simulink subsystem "decision_making"  (R2022b)
settings: Solver=VariableStepAuto  StartTime=0.0  StopTime=10.0  RelTol=1e-3
libraries: simulink x7, dspstat3 x4, slpidlib x1
settings Model: Creator=micha  LastModifiedBy=adter
settings ModelReferenceCC: EnableRefExpFcnMdlSchedulingChecks=on

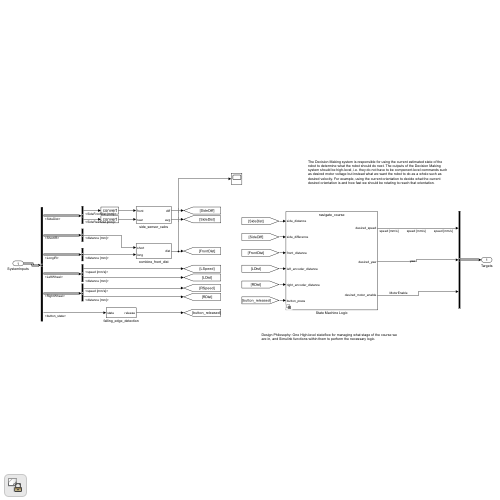
[thumbnail: Simulink's stored preview of the top-level diagram]
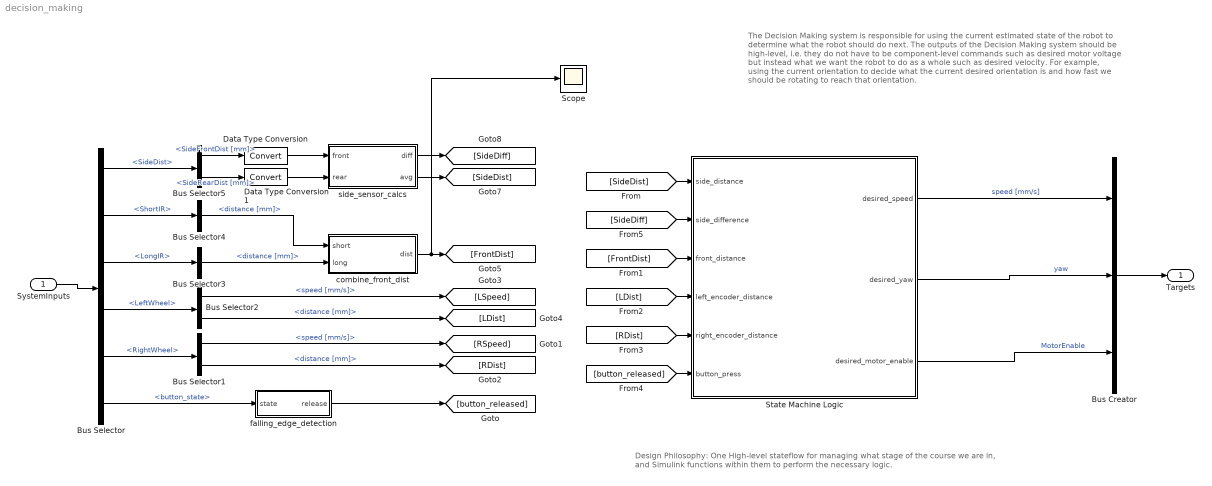
== system decision_making ==
  note: Design Philosophy: One High-level stateflow for managing what stage of the course we are in, and Simulink functions within them to perform the necessary logic.
  note: The Decision Making system is responsible for using the current estimated state of the robot to determine what the robot should do next. The outputs of the Decision Making system should be high-level, i.e. they do not have to be component-level commands such as desired motor voltage but instead what we want the robot to do as a whole such as desired velocity. For example, using the current orientation to decide what the current desired orientation is and how fast we should be rotating to reach that orientation.
  SystemInputs : Inport
  Bus Creator : BusCreator  Inputs=3
  Bus Selector : BusSelector  OutputSignals=SideDist,ShortIR,LongIR,LeftWheel,RightWheel,button.button_state
  Bus Selector1 : BusSelector  OutputSignals=speed [mm/s],distance [mm]
  Bus Selector2 : BusSelector  OutputSignals=speed [mm/s],distance [mm]
  Bus Selector3 : BusSelector  OutputSignals=distance [mm]
  Bus Selector4 : BusSelector  OutputSignals=distance [mm]
  Bus Selector5 : BusSelector  OutputSignals=SideFrontDist [mm],SideRearDist [mm]
  Data Type Conversion : DataTypeConversion  SaturateOnIntegerOverflow=off  RndMeth=Floor
  Data Type Conversion1 : DataTypeConversion  SaturateOnIntegerOverflow=off  RndMeth=Floor
  Scope : Scope
  State Machine Logic : Subsystem  Variant=on  VariantControlMode=label  LabelModeActiveChoice=true
  combine_front_dist : Subsystem
  falling_edge_detection : Subsystem
  side_sensor_calcs : Subsystem
  Targets : Outport
  wires:
  SystemInputs/1 -> Bus Selector/1
  State Machine Logic/2(desired_yaw) -> Bus Creator/2  "yaw"
  Bus Creator/1 -> Targets/1
  State Machine Logic/3(desired_motor_enable) -> Bus Creator/3  "MotorEnable"
  Bus Selector/6 -> falling_edge_detection/1(state)  "<button_state>"
  falling_edge_detection/1(release) -> [button_released]
  Bus Selector/5 -> Bus Selector1/1  "<RightWheel>"
  Bus Selector1/1 -> [RSpeed]  "<speed [mm/s]>"
  Bus Selector1/2 -> [RDist]  "<distance [mm]>"
  Bus Selector2/2 -> [LDist]  "<distance [mm]>"
  Bus Selector2/1 -> [LSpeed]  "<speed [mm/s]>"
  Bus Selector/4 -> Bus Selector2/1  "<LeftWheel>"
  Bus Selector/2 -> Bus Selector4/1  "<ShortIR>"
  Bus Selector/3 -> Bus Selector3/1  "<LongIR>"
  Bus Selector3/1 -> combine_front_dist/2(long)  "<distance [mm]>"
  Bus Selector4/1 -> combine_front_dist/1(short)  "<distance [mm]>"
  combine_front_dist/1(dist) -> [FrontDist], Scope/1
  [SideDist] -> State Machine Logic/1(side_distance)
  [FrontDist] -> State Machine Logic/3(front_distance)
  [LDist] -> State Machine Logic/4(left_encoder_distance)
  [RDist] -> State Machine Logic/5(right_encoder_distance)
  [button_released] -> State Machine Logic/6(button_press)
  State Machine Logic/1(desired_speed) -> Bus Creator/1  "speed [mm/s]"
  Bus Selector/1 -> Bus Selector5/1  "<SideDist>"
  Bus Selector5/2 -> Data Type Conversion1/1  "<SideRearDist [mm]>"
  Bus Selector5/1 -> Data Type Conversion/1  "<SideFrontDist [mm]>"
  side_sensor_calcs/2(avg) -> [SideDist]
  side_sensor_calcs/1(diff) -> [SideDiff]
  [SideDiff] -> State Machine Logic/2(side_difference)
  Data Type Conversion/1 -> side_sensor_calcs/1(front)
  Data Type Conversion1/1 -> side_sensor_calcs/2(rear)

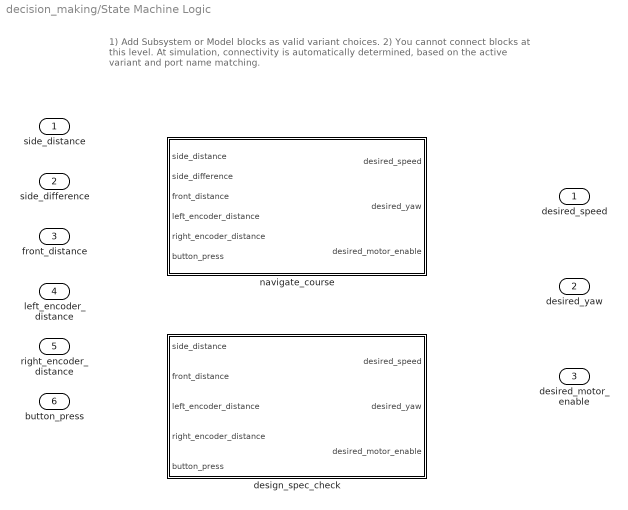
== system decision_making/State Machine Logic ==
  note: 1) Add Subsystem or Model blocks as valid variant choices.
      | 2) You cannot connect blocks at this level. At simulation, connectivity is automatically
      | determined, based on the active variant and port name matching.
  side_distance : Inport
  side_difference : Inport  Port=2
  front_distance : Inport  Port=3
  left_encoder_distance : Inport  Port=4
  right_encoder_distance : Inport  Port=5
  button_press : Inport  Port=6
  design_spec_check : Subsystem  VariantControl=false
  navigate_course : Subsystem  VariantControl=true
  desired_speed : Outport
  desired_yaw : Outport  Port=2
  desired_motor_enable : Outport  Port=3

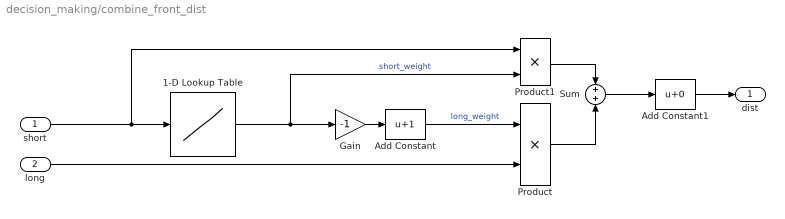
== system decision_making/combine_front_dist ==
  short : Inport
  long : Inport  Port=2
  1-D Lookup Table : Lookup_n-D  NumberOfTableDimensions=1  BreakpointsForDimension1=[0, 150, 300, 1000]  Table=[1, 1, 0, 0]  InternalRulePriority=Speed  RndMeth=Simplest
  Add Constant : Bias  Bias=1  SaturateOnIntegerOverflow=off
  Add Constant1 : Bias  SaturateOnIntegerOverflow=off
  Gain : Gain  Gain=-1
  Product : Product
  Product1 : Product
  Sum : Sum
  dist : Outport
  wires:
  Add Constant1/1 -> dist/1
  Sum/1 -> Add Constant1/1
  Product1/1 -> Sum/1
  Product/1 -> Sum/2
  long/1 -> Product/2
  Add Constant/1 -> Product/1  "long_weight"
  Gain/1 -> Add Constant/1
  1-D Lookup Table/1 -> Gain/1, Product1/2  "short_weight"
  short/1 -> 1-D Lookup Table/1, Product1/1

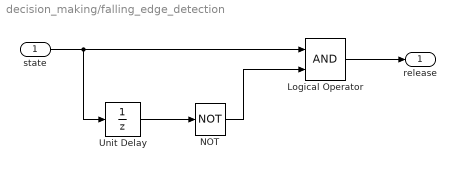
== system decision_making/falling_edge_detection ==
  state : Inport
  Logical Operator : Logic  IconShape=distinctive  AllPortsSameDT=off  OutDataTypeStr=boolean
  NOT : Logic  Operator=NOT  IconShape=distinctive  AllPortsSameDT=off  OutDataTypeStr=boolean
  Unit Delay : UnitDelay  SampleTime=-1  HasFrameUpgradeWarning=on
  release : Outport
  wires:
  NOT/1 -> Logical Operator/2
  state/1 -> Unit Delay/1, Logical Operator/1
  Logical Operator/1 -> release/1
  Unit Delay/1 -> NOT/1

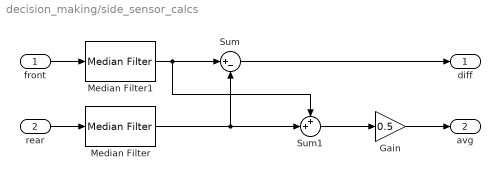
== system decision_making/side_sensor_calcs ==
  front : Inport
  rear : Inport  Port=2
  Gain : Gain  Gain=0.5
  Median Filter : dspstat3/Median Filter  WindowLength=5  SimulateUsing=Code generation
      settings: LibrarySourceBlock=|
      | dspfdesign/Median
      | Filter
  Median Filter1 : dspstat3/Median Filter  WindowLength=5  SimulateUsing=Code generation
      settings: LibrarySourceBlock=|
      | dspfdesign/Median
      | Filter
  Sum : Sum  Inputs=|+-
  Sum1 : Sum  Inputs=++|
  diff : Outport
  avg : Outport  Port=2
  wires:
  Median Filter1/1 -> Sum/1, Sum1/1
  Median Filter/1 -> Sum/2, Sum1/2
  Gain/1 -> avg/1
  Sum1/1 -> Gain/1
  Sum/1 -> diff/1
  rear/1 -> Median Filter/1
  front/1 -> Median Filter1/1

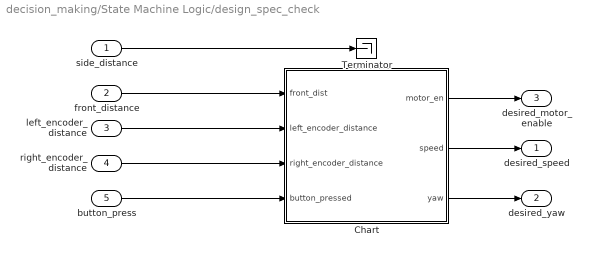
== system decision_making/State Machine Logic/design_spec_check ==
  side_distance : Inport
  front_distance : Inport  Port=2
  left_encoder_distance : Inport  Port=3
  right_encoder_distance : Inport  Port=4
  button_press : Inport  Port=5
  Chart : Stateflow chart  TreatAsAtomicUnit=on
  Terminator : Terminator
  desired_speed : Outport
  desired_yaw : Outport  Port=2
  desired_motor_enable : Outport  Port=3
  wires:
  button_press/1 -> Chart/4(button_pressed)
  front_distance/1 -> Chart/1(front_dist)
  right_encoder_distance/1 -> Chart/3(right_encoder_distance)
  left_encoder_distance/1 -> Chart/2(left_encoder_distance)
  side_distance/1 -> Terminator/1
  Chart/2(speed) -> desired_speed/1
  Chart/3(yaw) -> desired_yaw/1
  Chart/1(motor_en) -> desired_motor_enable/1

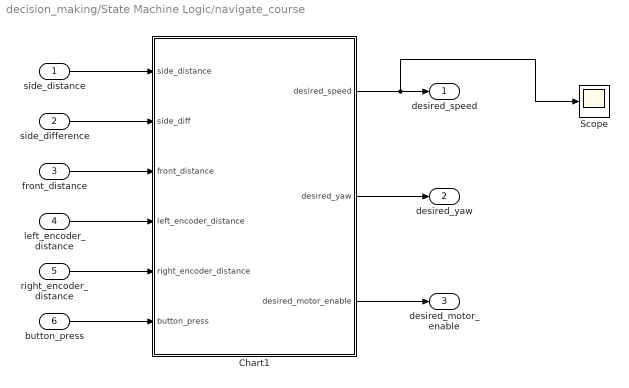
== system decision_making/State Machine Logic/navigate_course ==
  side_distance : Inport
  side_difference : Inport  Port=2
  front_distance : Inport  Port=3
  left_encoder_distance : Inport  Port=4
  right_encoder_distance : Inport  Port=5
  button_press : Inport  Port=6
  Chart1 : Stateflow chart  TreatAsAtomicUnit=on
  Scope : Scope
  desired_speed : Outport
  desired_yaw : Outport  Port=2
  desired_motor_enable : Outport  Port=3
  wires:
  side_difference/1 -> Chart1/2(side_diff)
  Chart1/3(desired_motor_enable) -> desired_motor_enable/1
  Chart1/2(desired_yaw) -> desired_yaw/1
  Chart1/1(desired_speed) -> desired_speed/1, Scope/1
  button_press/1 -> Chart1/6(button_press)
  right_encoder_distance/1 -> Chart1/5(right_encoder_distance)
  left_encoder_distance/1 -> Chart1/4(left_encoder_distance)
  front_distance/1 -> Chart1/3(front_distance)
  side_distance/1 -> Chart1/1(side_distance)

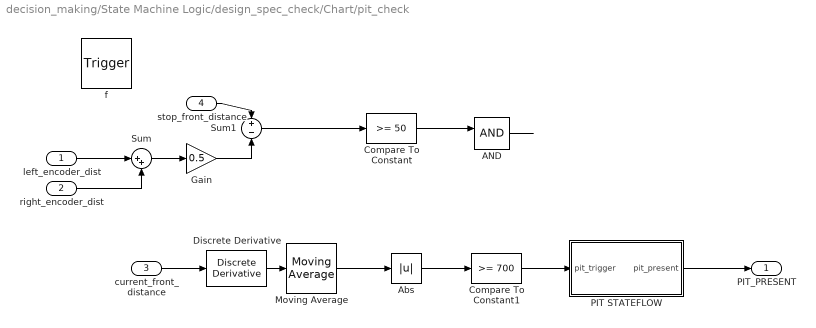
== system decision_making/State Machine Logic/design_spec_check/Chart/pit_check ==
  left_encoder_dist : Inport  OutDataTypeStr=int64  PortDimensions=1
  right_encoder_dist : Inport  Port=2  OutDataTypeStr=int64  PortDimensions=1
  current_front_distance : Inport  Port=3  OutDataTypeStr=double  PortDimensions=1
  stop_front_distance : Inport  Port=4  OutDataTypeStr=double  PortDimensions=1
  f : TriggerPort  TriggerType=function-call  VariantControl=(inherit)
      settings: CopyFcn=Stateflow.SLINSF.SimulinkMan.removeBlockPreDeleteFcn  PreDeleteFcn=Stateflow.SLINSF.SimulinkMan.unsafePredeleteFcn
  AND : Logic  IconShape=distinctive  AllPortsSameDT=off  OutDataTypeStr=boolean
  Abs : Abs  SaturateOnIntegerOverflow=off
  Compare To Constant : simulink/Logic and Bit Operations/Compare To Constant  relop=>=  const=50  OutDataTypeStr=boolean
  Compare To Constant1 : simulink/Logic and Bit Operations/Compare To Constant  relop=>=  const=700  OutDataTypeStr=boolean
  Discrete Derivative : simulink/Discrete/Discrete Derivative  gainval=1.0  ICPrevScaledInput=0.0  OutMin=[]  OutMax=[]  OutDataType=fixdt(1, 16)  OutScaling=2^-10  DoSatur=off
  Gain : Gain  Gain=0.5
  Moving Average : dspstat3/Moving Average  Method=Sliding window  ForgettingFactorPort=off  SpecifyWindowLength=on  WindowLength=50  OverlapLength=49  AllowArbitraryInputLength=off  ForgettingFactor=0.9  SimulateUsing=Code generation
  PIT STATEFLOW : Stateflow chart  TreatAsAtomicUnit=on
  Sum : Sum  Inputs=|++
  Sum1 : Sum  Inputs=+|-
  PIT_PRESENT : Outport  OutDataTypeStr=boolean
  wires:
  Abs/1 -> Compare To Constant1/1
  AND/1 -> ?
  PIT STATEFLOW/1(pit_present) -> PIT_PRESENT/1
  Compare To Constant/1 -> AND/1
  Moving Average/1 -> Abs/1
  Discrete Derivative/1 -> Moving Average/1
  Compare To Constant1/1 -> PIT STATEFLOW/1(pit_trigger)
  current_front_distance/1 -> Discrete Derivative/1
  Sum1/1 -> Compare To Constant/1
  Gain/1 -> Sum1/2
  stop_front_distance/1 -> Sum1/1
  Sum/1 -> Gain/1
  left_encoder_dist/1 -> Sum/1
  right_encoder_dist/1 -> Sum/2

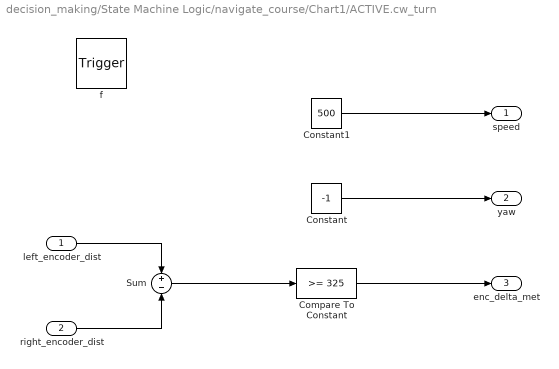
== system decision_making/State Machine Logic/navigate_course/Chart1/ACTIVE.cw_turn ==
  left_encoder_dist : Inport  OutDataTypeStr=int64  PortDimensions=1
  right_encoder_dist : Inport  Port=2  OutDataTypeStr=int64  PortDimensions=1
  f : TriggerPort  TriggerType=function-call  VariantControl=(inherit)
      settings: CopyFcn=Stateflow.SLINSF.SimulinkMan.removeBlockPreDeleteFcn  PreDeleteFcn=Stateflow.SLINSF.SimulinkMan.unsafePredeleteFcn
  Compare To Constant : simulink/Logic and Bit Operations/Compare To Constant  relop=>=  const=325  OutDataTypeStr=boolean
  Constant : Constant  Value=-1
  Constant1 : Constant  Value=500
  Sum : Sum  Inputs=+|-
  speed : Outport  OutDataTypeStr=double
  yaw : Outport  Port=2  OutDataTypeStr=double
  enc_delta_met : Outport  Port=3
  wires:
  Sum/1 -> Compare To Constant/1
  Compare To Constant/1 -> enc_delta_met/1
  right_encoder_dist/1 -> Sum/2
  left_encoder_dist/1 -> Sum/1
  Constant1/1 -> speed/1
  Constant/1 -> yaw/1

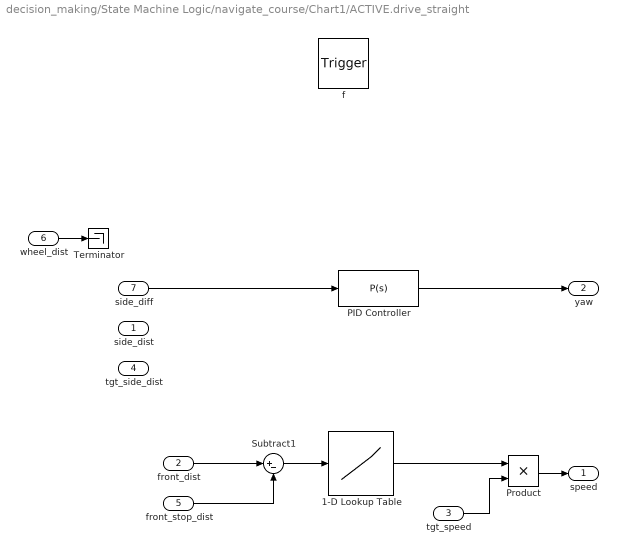
== system decision_making/State Machine Logic/navigate_course/Chart1/ACTIVE.drive_straight ==
  side_dist : Inport  OutDataTypeStr=double  PortDimensions=1
  front_dist : Inport  Port=2  OutDataTypeStr=double  PortDimensions=1
  tgt_speed : Inport  Port=3  OutDataTypeStr=double  PortDimensions=1
  tgt_side_dist : Inport  Port=4  OutDataTypeStr=double  PortDimensions=1
  front_stop_dist : Inport  Port=5  OutDataTypeStr=double  PortDimensions=1
  wheel_dist : Inport  Port=6  OutDataTypeStr=int64  PortDimensions=1
  side_diff : Inport  Port=7  OutDataTypeStr=double  PortDimensions=1
  f : TriggerPort  TriggerType=function-call  VariantControl=(inherit)  SampleTimeType=periodic  SampleTime=(-1)
      settings: CopyFcn=Stateflow.SLINSF.SimulinkMan.removeBlockPreDeleteFcn  PreDeleteFcn=Stateflow.SLINSF.SimulinkMan.unsafePredeleteFcn
  1-D Lookup Table : Lookup_n-D  NumberOfTableDimensions=1  BreakpointsForDimension1=[0,150,2000]  Table=[0.1,1,1]  ExtrapMethod=Clip  UseLastTableValue=on  InternalRulePriority=Speed  RndMeth=Simplest
  PID Controller : slpidlib/PID Controller  Controller=P  Form=Parallel  TimeDomain=Continuous-time  UseExternalTs=off  SampleTime=-1  IntegratorMethod=Forward Euler  FilterMethod=Forward Euler  ControllerParametersSource=internal  P=0.25/20  I=1  UseKiTs=off  D=0  N=100  UseFilter=on  TunerSelectOption=Transfer Function Based (PID Tuner App)  InitialConditionSource=internal  InitialConditionForIntegrator=0  InitialConditionForFilter=0  DifferentiatorICPrevScaledInput=0  ExternalReset=none  TrackingMode=off  Kt=1  LimitOutput=on  SatLimitsSource=internal  UpperSaturationLimit=0.25  LowerSaturationLimit=-0.25  LinearizeAsGain=on  AntiWindupMode=none  Kb=1  LimitIntegrator=off  UpperIntegratorSaturationLimit=inf  LowerIntegratorSaturationLimit=-inf  POutMin=[]  POutMax=[]  IOutMin=[]  IOutMax=[]  DOutMin=[]  DOutMax=[]  NOutMin=[]  NOutMax=[]  SumOutMin=[]  SumOutMax=[]  SaturationOutMin=[]  SaturationOutMax=[]  PParamMin=[]  PParamMax=[]  IParamMin=[]  IParamMax=[]  DParamMin=[]  DParamMax=[]  NParamMin=[]  NParamMax=[]  KbParamMin=[]  KbParamMax=[]  KtParamMin=[]  KtParamMax=[]  KbOutMin=[]  KbOutMax=[]  KtOutMin=[]  KtOutMax=[]  IntegratorOutMin=[]  IntegratorOutMax=[]  FilterOutMin=[]  FilterOutMax=[]  SumI1OutMin=[]  SumI1OutMax=[]  SumI2OutMin=[]  SumI2OutMax=[]  SumI3OutMin=[]  SumI3OutMax=[]  SumI4OutMin=[]  SumI4OutMax=[]  SumDOutMin=[]  SumDOutMax=[]  DifferentiatorOutMin=[]  DifferentiatorOutMax=[]  FilterDiffOutCoefMin=[]  FilterDiffOutCoefMax=[]  ReciprocalOutMin=[]  ReciprocalOutMax=[]  SumDenOutMin=[]  SumDenOutMax=[]  SumNumOutMin=[]  SumNumOutMax=[]  DivideOutMin=[]  DivideOutMax=[]  UdiffTsProdOutMin=[]  UdiffTsProdOutMax=[]  NTsProdOutMin=[]  NTsProdOutMax=[]  UintegralTsProdOutMin=[]  UintegralTsProdOutMax=[]  UngainTsProdOutMin=[]  UngainTsProdOutMax=[]  ClampingZeroOutDataTypeStr=Inherit: Inherit via back propagation  ClampingZeroOutMin=[]  ClampingZeroOutMax=[]  FilterDenConstantOutDataTypeStr=Inherit: Inherit via back propagation  FilterDenConstantOutMin=[]  FilterDenConstantOutMax=[]  PCopyOutDataTypeStr=Inherit: Inherit via back propagation  PCopyOutMin=[]  PCopyOutMax=[]  NCopyOutDataTypeStr=Inherit: Inherit via back propagation  NCopyOutMin=[]  NCopyOutMax=[]  IntegratorContinuousStateAttributes=''  IntegratorStateMustResolveToSignalObject=off  IntegratorRTWStateStorageClass=Auto  FilterContinuousStateAttributes=''  FilterStateMustResolveToSignalObject=off  FilterRTWStateStorageClass=Auto  ParallelPVariant=InternalParameters  IdealPVariant=Disabled  IVariant=Disabled  DVariant=Disabled  IntegratorVariant=Disabled  SatVariant=Enabled  AWVariant=Disabled  PCopyVariant=Disabled  TRVariant=Disabled  FdbkBlocksVariant=Forward  IdealPFdbkVariant=Disabled  SatFdbkVariant=Disabled  DerivativeFilterVariant=Disabled  NVariant=Disabled  NCopyVariant=Disabled_SignalSpec  FilterICVariant=Disabled  IntegratorICVariant=Disabled  ExternalResetVariant=Disabled  TRSumVariant=Passthrough  SumFdbkVariant=Disabled  SumVariant=Passthrough_P  TsampFilterVariant=InternalTs  TsampNgainVariant=Passthrough  TsampIntegralVariant=Disabled_SignalSpec  ExternalSaturationOutDataTypeStr=Inherit: Same as second input
  Product : Product
  Subtract1 : Sum  Inputs=|+-
  Terminator : Terminator
  speed : Outport
  yaw : Outport  Port=2
  wires:
  PID Controller/1 -> yaw/1
  side_diff/1 -> PID Controller/1
  Product/1 -> speed/1
  wheel_dist/1 -> Terminator/1
  tgt_speed/1 -> Product/2
  1-D Lookup Table/1 -> Product/1
  front_stop_dist/1 -> Subtract1/2
  front_dist/1 -> Subtract1/1
  Subtract1/1 -> 1-D Lookup Table/1

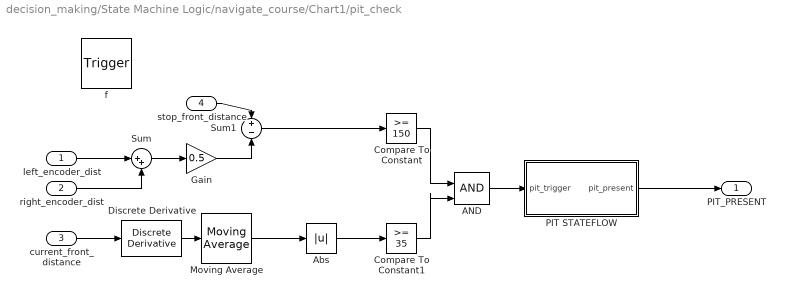
== system decision_making/State Machine Logic/navigate_course/Chart1/pit_check ==
  left_encoder_dist : Inport  OutDataTypeStr=int64  PortDimensions=1
  right_encoder_dist : Inport  Port=2  OutDataTypeStr=int64  PortDimensions=1
  current_front_distance : Inport  Port=3  OutDataTypeStr=double  PortDimensions=1
  stop_front_distance : Inport  Port=4  OutDataTypeStr=double  PortDimensions=1
  f : TriggerPort  TriggerType=function-call  VariantControl=(inherit)
      settings: CopyFcn=Stateflow.SLINSF.SimulinkMan.removeBlockPreDeleteFcn  PreDeleteFcn=Stateflow.SLINSF.SimulinkMan.unsafePredeleteFcn
  AND : Logic  IconShape=distinctive  AllPortsSameDT=off  OutDataTypeStr=boolean
  Abs : Abs  SaturateOnIntegerOverflow=off
  Compare To Constant : simulink/Logic and Bit Operations/Compare To Constant  relop=>=  const=150  OutDataTypeStr=boolean
  Compare To Constant1 : simulink/Logic and Bit Operations/Compare To Constant  relop=>=  const=35  OutDataTypeStr=boolean
  Discrete Derivative : simulink/Discrete/Discrete Derivative  gainval=1.0  ICPrevScaledInput=0.0  OutMin=[]  OutMax=[]  OutDataType=fixdt(1, 16)  OutScaling=2^-10  DoSatur=off
  Gain : Gain  Gain=0.5
  Moving Average : dspstat3/Moving Average  Method=Sliding window  ForgettingFactorPort=off  SpecifyWindowLength=on  WindowLength=50  OverlapLength=49  AllowArbitraryInputLength=off  ForgettingFactor=0.9  SimulateUsing=Code generation
  PIT STATEFLOW : Stateflow chart  TreatAsAtomicUnit=on
  Sum : Sum  Inputs=|++
  Sum1 : Sum  Inputs=+|-
  PIT_PRESENT : Outport  OutDataTypeStr=boolean
  wires:
  Abs/1 -> Compare To Constant1/1
  AND/1 -> PIT STATEFLOW/1(pit_trigger)
  PIT STATEFLOW/1(pit_present) -> PIT_PRESENT/1
  Compare To Constant/1 -> AND/1
  Moving Average/1 -> Abs/1
  Discrete Derivative/1 -> Moving Average/1
  Compare To Constant1/1 -> AND/2
  current_front_distance/1 -> Discrete Derivative/1
  Sum1/1 -> Compare To Constant/1
  Gain/1 -> Sum1/2
  stop_front_distance/1 -> Sum1/1
  Sum/1 -> Gain/1
  left_encoder_dist/1 -> Sum/1
  right_encoder_dist/1 -> Sum/2

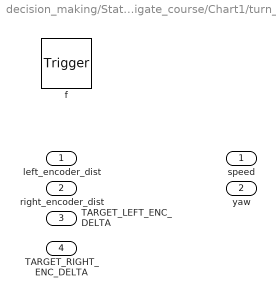
== system decision_making/State Machine Logic/navigate_course/Chart1/turn_zero ==
  left_encoder_dist : Inport  OutDataTypeStr=double  PortDimensions=1
  right_encoder_dist : Inport  Port=2  OutDataTypeStr=double  PortDimensions=1
  TARGET_LEFT_ENC_DELTA : Inport  Port=3  OutDataTypeStr=double  PortDimensions=1
  TARGET_RIGHT_ENC_DELTA : Inport  Port=4  OutDataTypeStr=double  PortDimensions=1
  f : TriggerPort  TriggerType=function-call  VariantControl=(inherit)
      settings: CopyFcn=Stateflow.SLINSF.SimulinkMan.removeBlockPreDeleteFcn  PreDeleteFcn=Stateflow.SLINSF.SimulinkMan.unsafePredeleteFcn
  speed : Outport
  yaw : Outport  Port=2

== stateflow chart decision_making/State Machine Logic/navigate_course/Chart1/pit_check/PIT STATEFLOW ==
  state OUT_OF_PIT
    en: pit_present = false;
  state IN_PIT
    en: pit_present = true;
    en: pit_time = et;
  (default) -> OUT_OF_PIT
  IN_PIT -> OUT_OF_PIT : [pit_trigger == true && (pit_time - et) > 0.5]
  OUT_OF_PIT -> IN_PIT : [pit_trigger == true]
  data: pit_trigger input boolean; pit_present output boolean =false; pit_time local =0

== stateflow chart decision_making/State Machine Logic/design_spec_check/Chart ==
  state IDLE
    en, du: motor_en = false;
    en, du: speed = 0;
    en, du: yaw = 0;
    du: [pit_detected] = pit_check(left_encoder_distance, right_encoder_distance, front_dist, STOP_DIST);
  state PIT_PRESENT  = pit_check(left_encoder_dist,right_encoder_dist, current_front_distance, stop_front_distance) [function]
  state TEST1
    en, du: motor_en = true;
    en, du: yaw = 0;
    en, du: speed = 600;
    du: [pit_detected] = pit_check(left_encoder_distance, right_encoder_distance, front_dist, STOP_DIST);
  state TEST3
    en, du: motor_en = true;
    en, du: yaw = 0;
    en, du: speed = 200;
    du: [pit_detected] = pit_check(left_encoder_distance, right_encoder_distance, front_dist, STOP_DIST);
  (default) -> IDLE
  TEST3 -> IDLE : [button_pressed || front_dist <= STOP_DIST]
  TEST1 -> IDLE [order 1] : [button_pressed || front_dist <= STOP_DIST]
  IDLE -> TEST1 : [button_pressed]
  TEST1 -> TEST3 [order 2] : [pit_detected]
  data: left_encoder_dist function_input int64 size=1; right_encoder_dist function_input int64 size=1; PIT_PRESENT function_output boolean; current_front_distance function_input double size=1; stop_front_distance function_input double size=1; motor_en output boolean; speed output; yaw output; STOP_DIST constant double =100; front_dist input; left_encoder_distance input; right_encoder_distance input; button_pressed input boolean; pit_detected local

== stateflow chart decision_making/State Machine Logic/navigate_course/Chart1 ==
  state PIT_PRESENT  = pit_check(left_encoder_dist,right_encoder_dist, current_front_distance, stop_front_distance) [function] [commented out]
  state IDLE
    en: desired_speed = 0;
    en: desired_yaw = 0;
    en: desired_motor_enable = false;
  state [speed, yaw] =   turn_zero(left_encoder_dist, right_encoder_dist, TARGET_LEFT_ENC_DELTA, TARGET_RIGHT_ENC_DELTA) [function] [commented out]
  state ACTIVE
    en: desired_motor_enable = true;
    state [speed,yaw] = drive_straight(side_dist,front_dist,tgt_speed,tgt_side_dist,front_stop_dist,wheel_dist,side_diff) [function]
    state [speed,yaw,enc_delta_met] = cw_turn(left_encoder_dist,right_encoder_dist) [function]
    state STAGE_0_DRIVE
      en: left_eref = left_encoder_distance;
      en: right_eref = right_encoder_distance;
      en,during: [desired_speed, desired_yaw] = drive_straight(side_distance, front_distance, TARGET_SPEED, OUTER_LOOP_SIDE_DIST,...
      OUTER_LOOP_FRONT_STOP_DIST, ((left_encoder_distance - left_eref) + (right_encoder_distance - right_eref))/2, side_diff);
    state STAGE_0_TURN
      en: ENC_DELTAS_MET = false;
      en: left_eref = left_encoder_distance;
      en: right_eref = right_encoder_distance;
      en: in_pit = false;
      du: [desired_speed, desired_yaw, ENC_DELTAS_MET] = cw_turn((left_encoder_distance - left_eref), (right_encoder_distance - right_eref));
    state STAGE_1_DRIVE
      en: left_eref = left_encoder_distance;
      en: right_eref = right_encoder_distance;
      en,during: [desired_speed, desired_yaw] = drive_straight(side_distance, front_distance, TARGET_SPEED, OUTER_LOOP_SIDE_DIST,...
      OUTER_LOOP_FRONT_STOP_DIST, ((left_encoder_distance - left_eref) + (right_encoder_distance - right_eref))/2, side_diff);
    state STAGE_1_TURN
      en: ENC_DELTAS_MET = false;
      en: left_eref = left_encoder_distance;
      en: right_eref = right_encoder_distance;
      en: in_pit = false;
      du: [desired_speed, desired_yaw, ENC_DELTAS_MET] = cw_turn((left_encoder_distance - left_eref), (right_encoder_distance - right_eref));
    state STAGE_2_DRIVE
      en: left_eref = left_encoder_distance;
      en: right_eref = right_encoder_distance;
      en,during: [desired_speed, desired_yaw] = drive_straight(side_distance, front_distance, TARGET_SPEED, OUTER_LOOP_SIDE_DIST,...
      OUTER_LOOP_FRONT_STOP_DIST, ((left_encoder_distance - left_eref) + (right_encoder_distance - right_eref))/2, side_diff);
    state STAGE_2_TURN
      en: ENC_DELTAS_MET = false;
      en: left_eref = left_encoder_distance;
      en: right_eref = right_encoder_distance;
      en: in_pit = false;
      du: [desired_speed, desired_yaw, ENC_DELTAS_MET] = cw_turn((left_encoder_distance - left_eref), (right_encoder_distance - right_eref));
    state STAGE_3_DRIVE
      en: left_eref = left_encoder_distance;
      en: right_eref = right_encoder_distance;
      en,during: [desired_speed, desired_yaw] = drive_straight(side_distance, front_distance, TARGET_SPEED, MIDDLE_LOOP_SIDE_DIST,...
      MIDDLE_LOOP_FRONT_STOP_DIST, ((left_encoder_distance - left_eref) + (right_encoder_distance - right_eref))/2, side_diff);
    state STAGE_3_TURN
      en: ENC_DELTAS_MET = false;
      en: left_eref = left_encoder_distance;
      en: right_eref = right_encoder_distance;
      en: in_pit = false;
      du: [desired_speed, desired_yaw, ENC_DELTAS_MET] = cw_turn((left_encoder_distance - left_eref), (right_encoder_distance - right_eref));
    (default) -> STAGE_0_DRIVE
    STAGE_0_DRIVE -> STAGE_0_TURN [order 1] : [front_distance <= OUTER_LOOP_FRONT_STOP_DIST &&...
        | ((left_encoder_distance - left_eref) + (right_encoder_distance - right_eref))/2 > 500]
    STAGE_0_TURN -> STAGE_1_DRIVE : [ENC_DELTAS_MET]
    STAGE_1_DRIVE -> STAGE_1_TURN : [front_distance <= OUTER_LOOP_FRONT_STOP_DIST &&...
        | ((left_encoder_distance - left_eref) + (right_encoder_distance - right_eref))/2 > 500]
    STAGE_1_TURN -> STAGE_2_DRIVE : [ENC_DELTAS_MET]
    STAGE_2_DRIVE -> STAGE_2_TURN : [front_distance <= OUTER_LOOP_FRONT_STOP_DIST &&...
        | ((left_encoder_distance - left_eref) + (right_encoder_distance - right_eref))/2 > 500]
    STAGE_2_TURN -> STAGE_3_DRIVE : [ENC_DELTAS_MET]
    STAGE_3_DRIVE -> STAGE_3_TURN : [front_distance <= MIDDLE_LOOP_FRONT_STOP_DIST &&...
        | ((left_encoder_distance - left_eref) + (right_encoder_distance - right_eref))/2 > 800]
  (default) -> IDLE
  STAGE_0_DRIVE -> IDLE [order 2] : [((left_encoder_distance - left_eref) + (right_encoder_distance - right_eref))/2 > 3000]
  STAGE_3_TURN -> IDLE : [ENC_DELTAS_MET]
  ACTIVE -> IDLE : [button_press]
  IDLE -> ACTIVE : [button_press]
  data: left_encoder_dist function_input double size=1; right_encoder_dist function_input double size=1; PIT_PRESENT function_output double size=1; current_front_distance function_input double size=1; stop_front_distance function_input double size=1; left_encoder_dist function_input double size=1; right_encoder_dist function_input double size=1; speed function_output double size=1; yaw function_output double size=1; TARGET_LEFT_ENC_DELTA function_input double size=1; TARGET_RIGHT_ENC_DELTA function_input double size=1; speed function_output; side_dist function_input double size=1; front_dist function_input double size=1; yaw function_output; tgt_speed function_input double size=1; tgt_side_dist function_input double size=1; front_stop_dist function_input double size=1; wheel_dist function_input int64 size=1; side_diff function_input double size=1; left_encoder_dist function_input int64 size=1; right_encoder_dist function_input int64 size=1; speed function_output double; yaw function_output double; enc_delta_met function_output; desired_speed output double =0; desired_yaw output double [-1..1] =0; desired_motor_enable output boolean; side_distance input; side_diff input; front_distance input; left_encoder_distance input; right_encoder_distance input size=1; button_press input boolean; OUTER_LOOP_SIDE_DIST constant double =75; OUTER_LOOP_FRONT_STOP_DIST constant double =135; TARGET_SPEED constant double =400; WHEEL_DIAMETER constant double =95; TURN_ANGLE constant double =90; APPROACHING_SPEED constant double =150; MIDDLE_LOOP_SIDE_DIST constant double =250; MIDDLE_LOOP_FRONT_STOP_DIST constant double =470; INNER_LOOP_SIDE_DIST constant double =350; INNER_LOOP_FRONT_STOP_DIST constant double =350; ENC_DELTAS_MET local boolean =false; IDEAL_RIGHT_ENC_DELTA constant double =(pi()/2)*25; IDEAL_LEFT_ENC_DELTA constant double =(pi()/2)*185; left_eref local int64 =int64(0); right_eref local int64 =int64(0); in_pit local boolean =false

== stateflow chart decision_making/State Machine Logic/design_spec_check/Chart/pit_check/PIT STATEFLOW ==
  state OUT_OF_PIT
    en: pit_present = false;
  state IN_PIT
    en: pit_present = true;
  (default) -> OUT_OF_PIT
  IN_PIT -> OUT_OF_PIT [order 1] : [et > 1]
  OUT_OF_PIT -> IN_PIT : [pit_trigger && et > 1.5]
  IN_PIT -> OUT_OF_PIT [order 2] : [et > 10]
  data: pit_trigger input boolean; pit_present output boolean =false; pit_time local =0
